simulink model "Validation_Tricopter_Model"  (R2015a)
settings: Solver=ode3  SolverMode=SingleTasking  StartTime=0.0  StopTime=20  FixedStep=T_sim  RelTol=1e-3
PreLoadFcn:
  | LoadLibraries
values from neighbouring files (symbols this model uses):
  a = 10.26    [SetupComplete.m]
  A_x = 0.015    [SetupComplete.m]
  A_y = A_x    (= 0.015)    [SetupComplete.m]
  A_z = 0.16    [SetupComplete.m]
  C_d0 = 0.001193    [SetupComplete.m]
  C_x = 1.2    [SetupComplete.m]
  C_y = C_x    (= 1.2)    [SetupComplete.m]
  C_z = 2.2    [SetupComplete.m]
  CG_0 = [0,0,0.02]'    [SetupComplete.m]
  g = 9.81    [SetupComplete.m]
  h = 0.08    [SetupComplete.m]
  h_FA = 0.02    [SetupComplete.m]
  h_M = 0.064    [SetupComplete.m]
  I_BAC_0 = [ Ix,0,Ixz;0,Iy,0;Ixz,0,Iz]    [SetupComplete.m]
  I_prop = 1/4*M_eq*R^2*diag([1,1,2])    [SetupComplete.m]
  I_tube = [1/2*M_tube*R_tube_eq^2,0,  0  ;           0 ,1/3*M_tube*l_arm^2,0;             0  ,0,1/3*M_tube*l_arm^2]    [SetupComplete.m]
  Initial_Omegas = [1;1;1]*Omega_hover    [Run3Copter.m]
  J_FA = I_prop(1,1) + m_prop*h^2  + m_FA*h_FA^2 + m_M*h_M^2    [SetupComplete.m]
  J_T = J_m+1/2*M_eq*R^2    (= 2.000642e-05)    [SetupComplete.m]
  Ki = lqi(LM_4DOF_aug, Q,R)    [robust_controller.m]
  l = 0.3450    (= 0.345)    [NDI_components.m]    (also in SetupComplete.m; robust_controller.m)
  l_arm = 0.264    [SetupComplete.m]
  m = 3.51    [SetupComplete.m]
  m_0 = 2.61    [SetupComplete.m]
  m_FA = 0.02    [SetupComplete.m]
  m_M = 0.300    (= 0.3)    [SetupComplete.m]
  m_prop = 0.02    [SetupComplete.m]
  R = 0.1778    [SetupComplete.m]    (also in robust_controller.m = eye(4))
  rho = 1.15    [SetupComplete.m]
  sigma = b*c/(pi*R)    (= 0.107416159567)    [SetupComplete.m]
  T_sim = 0.01    [Run3Copter.m]
  theta_0 = 0.38397    [SetupComplete.m]
  theta_1 = -0.2967    [SetupComplete.m]
  trim_simplemodel = [0.589627915568 -2.20656039197 0 0.588313336084 0 0 0.588313330414 0 0]    [trimvalues.mat]
  V_4DOF_last = [0.0122475086001 0.00870447045314 -0.0292257707267 -0.0198753669721 -0.00290766514824 -0.0269511839788 0.0344308792695 -0.0305235710433 -0.0274078219028 -0.0329291952852 -0.0272335702183 -0.00643013158961 ... (1500 elements, 50x30)]    [NN_c_weights.mat]
  v_i0 = sqrt( 1/3*m*g/(2*rho*pi*R^2)  )    [SetupComplete.m]
  W_4DOF_last = [0.0132359246225 -0.0402459595001 -0.0221501781133 0.0046881519205 0.0457506835434 0.0464888535199 -0.0342386918322 0.0470592781761 0.0457166948243 -0.00146243512772 0.0300280468889 -0.0358113661373 ... (204 elements, 4x51)]    [NN_c_weights.mat]
undefined symbols (not defined in the file or in its folder): DOWN_0, EAST_0, Motor, NORTH_0, P_0, Prop, Q_0, R_0, sigmatest, U_0, V_0, v_i_adim, Vx_adim, Vz_adim, W_0
undefined symbols (not defined in the file): Initial_Torques, Rotation_sign, Tau_motors
libraries: simulink x66, XXCopter x32, vrlib x26, simulink_extras x6, Adaptive_FaultTolerantControl x6, qcatlib x4, dspinverses x4, lib_controller x4, aerolib6dofsys x3, aerolibtransform2 x3, aerolib6dof2 x1
(part 2 of 11)

== system Validation_Tricopter_Model/Controller/4DOF PID Controller/4DOF PI Angle Controller ==
  note: This DCM is Tb->e
      | Xbody = DCM x Xearth
  note: Proportional controller around the hovering point. Body rates will be very similar to euler rates.
  note: INNER RATE LOOP TUNING
  note: INNER ANGLE LOOP TUNING
  measurements : Inport
  earth_ref : Inport  Port=2
  trim_control_input : Inport  Port=3
  Reference_attitude : Inport  Port=4
  Bus Selector : BusSelector  OutputSignals=euler,euler_dot,X_e,DCM,V_b
  Demux{,1,3..8} (8 alike) : Demux  Outputs=3
  Earth to body : Product  Multiplication=Matrix(*)
  Inner Rate Controller1 : ModelReference  ModelNameDialog=Inner_Rate_Controller  SimulationMode=Normal  ModelReferenceVersion=1.1241  CopyOfModelName=Inner_Rate_Controller
  Mux1 : Mux  Inputs=3
  Mux2 : Mux  Inputs=3
  Mux3 : Mux  Inputs=3
  PID Controller : simulink/Continuous/PID Controller  Controller=PI  TimeDomain=Continuous-time  SampleTime=-1  IntegratorMethod=Forward Euler  FilterMethod=Forward Euler  Form=Parallel  UseFilter=on  ControllerParametersSource=internal  P=1  I=1  D=0  N=100  InitialConditionSource=internal  InitialConditionForIntegrator=0  InitialConditionForFilter=0  ExternalReset=none  LimitOutput=off  UpperSaturationLimit=inf  LowerSaturationLimit=-inf  LinearizeAsGain=on  AntiWindupMode=none  Kb=1  TrackingMode=off  Kt=1  PParamMin=[]  PParamMax=[]  IParamMin=[]  IParamMax=[]  DParamMin=[]  DParamMax=[]  NParamMin=[]  NParamMax=[]  KbParamMin=[]  KbParamMax=[]  KtParamMin=[]  KtParamMax=[]  POutMin=[]  POutMax=[]  IOutMin=[]  IOutMax=[]  DOutMin=[]  DOutMax=[]  NOutMin=[]  NOutMax=[]  KbOutMin=[]  KbOutMax=[]  KtOutMin=[]  KtOutMax=[]  IntegratorOutMin=[]  IntegratorOutMax=[]  FilterOutMin=[]  FilterOutMax=[]  SumOutMin=[]  SumOutMax=[]  SumI1OutMin=[]  SumI1OutMax=[]  SumI2OutMin=[]  SumI2OutMax=[]  SumI3OutMin=[]  SumI3OutMax=[]  SumDOutMin=[]  SumDOutMax=[]  SaturationOutMin=[]  SaturationOutMax=[]  IntegratorContinuousStateAttributes=''  IntegratorStateMustResolveToSignalObject=off  IntegratorRTWStateStorageClass=Auto  FilterContinuousStateAttributes=''  FilterStateMustResolveToSignalObject=off  FilterRTWStateStorageClass=Auto  DifferentiatorICPrevScaledInput=0  DifferentiatorOutMin=[]  DifferentiatorOutMax=[]
  PID Controller1 : simulink/Continuous/PID Controller  Controller=PI  TimeDomain=Continuous-time  SampleTime=-1  IntegratorMethod=Forward Euler  FilterMethod=Forward Euler  Form=Parallel  UseFilter=on  ControllerParametersSource=internal  P=1  I=1  D=0  N=100  InitialConditionSource=internal  InitialConditionForIntegrator=0  InitialConditionForFilter=0  ExternalReset=none  LimitOutput=off  UpperSaturationLimit=inf  LowerSaturationLimit=-inf  LinearizeAsGain=on  AntiWindupMode=none  Kb=1  TrackingMode=off  Kt=1  PParamMin=[]  PParamMax=[]  IParamMin=[]  IParamMax=[]  DParamMin=[]  DParamMax=[]  NParamMin=[]  NParamMax=[]  KbParamMin=[]  KbParamMax=[]  KtParamMin=[]  KtParamMax=[]  POutMin=[]  POutMax=[]  IOutMin=[]  IOutMax=[]  DOutMin=[]  DOutMax=[]  NOutMin=[]  NOutMax=[]  KbOutMin=[]  KbOutMax=[]  KtOutMin=[]  KtOutMax=[]  IntegratorOutMin=[]  IntegratorOutMax=[]  FilterOutMin=[]  FilterOutMax=[]  SumOutMin=[]  SumOutMax=[]  SumI1OutMin=[]  SumI1OutMax=[]  SumI2OutMin=[]  SumI2OutMax=[]  SumI3OutMin=[]  SumI3OutMax=[]  SumDOutMin=[]  SumDOutMax=[]  SaturationOutMin=[]  SaturationOutMax=[]  IntegratorContinuousStateAttributes=''  IntegratorStateMustResolveToSignalObject=off  IntegratorRTWStateStorageClass=Auto  FilterContinuousStateAttributes=''  FilterStateMustResolveToSignalObject=off  FilterRTWStateStorageClass=Auto  DifferentiatorICPrevScaledInput=0  DifferentiatorOutMin=[]  DifferentiatorOutMax=[]
  PID Controller2 : simulink/Continuous/PID Controller  Controller=PI  TimeDomain=Continuous-time  SampleTime=-1  IntegratorMethod=Forward Euler  FilterMethod=Forward Euler  Form=Parallel  UseFilter=on  ControllerParametersSource=internal  P=1  I=0.1  D=0  N=100  InitialConditionSource=internal  InitialConditionForIntegrator=0  InitialConditionForFilter=0  ExternalReset=none  LimitOutput=off  UpperSaturationLimit=inf  LowerSaturationLimit=-inf  LinearizeAsGain=on  AntiWindupMode=none  Kb=1  TrackingMode=off  Kt=1  PParamMin=[]  PParamMax=[]  IParamMin=[]  IParamMax=[]  DParamMin=[]  DParamMax=[]  NParamMin=[]  NParamMax=[]  KbParamMin=[]  KbParamMax=[]  KtParamMin=[]  KtParamMax=[]  POutMin=[]  POutMax=[]  IOutMin=[]  IOutMax=[]  DOutMin=[]  DOutMax=[]  NOutMin=[]  NOutMax=[]  KbOutMin=[]  KbOutMax=[]  KtOutMin=[]  KtOutMax=[]  IntegratorOutMin=[]  IntegratorOutMax=[]  FilterOutMin=[]  FilterOutMax=[]  SumOutMin=[]  SumOutMax=[]  SumI1OutMin=[]  SumI1OutMax=[]  SumI2OutMin=[]  SumI2OutMax=[]  SumI3OutMin=[]  SumI3OutMax=[]  SumDOutMin=[]  SumDOutMax=[]  SaturationOutMin=[]  SaturationOutMax=[]  IntegratorContinuousStateAttributes=''  IntegratorStateMustResolveToSignalObject=off  IntegratorRTWStateStorageClass=Auto  FilterContinuousStateAttributes=''  FilterStateMustResolveToSignalObject=off  FilterRTWStateStorageClass=Auto  DifferentiatorICPrevScaledInput=0  DifferentiatorOutMin=[]  DifferentiatorOutMax=[]
  Sum : Sum  Inputs=|+-
  Sum1 : Sum  Inputs=-+|
  Sum2 : Sum  Inputs=|++
  Sum3 : Sum  Inputs=-+|
  Sum4 : Sum  Inputs=|+-
  euler_ref : Constant  Value=[0,0,0]
  Controller output : Outport
  wires:
  [psi_error] -> PID Controller2/1
  [theta_error] -> PID Controller1/1
  PID Controller2/1 -> [r_ref]
  PID Controller1/1 -> [q_ref]
  PID Controller/1 -> [p_ref]
  [phi_error] -> PID Controller/1
  Demux3/3 -> [r]
  Demux3/2 -> [q]
  Demux3/1 -> [p]
  measurements/1 -> Bus Selector/1
  Sum2/1 -> Controller output/1
  Bus Selector/2 -> Demux3/1, Sum1/1  "<euler_dot>"
  Sum1/1 -> Demux/1
  Demux/3 -> [r_error]
  Demux/2 -> [q_error]
  Demux/1 -> [p_error]
  trim_control_input/1 -> [trimmed_input]
  [trimmed_input] -> Sum2/2
  Mux2/1 -> Sum1/2
  [q_ref] -> Mux2/2
  [p_ref] -> Mux2/1
  [r_ref] -> Mux2/3
  Inner Rate Controller1/1 -> Sum2/1
  [p_error] -> Inner Rate Controller1/1
  [q_error] -> Inner Rate Controller1/2
  [r_error] -> Inner Rate Controller1/3
  Bus Selector/3 -> Demux5/1, Sum3/1  "<X_e>"
  Demux5/3 -> [Z_earth]
  Demux5/2 -> [Y_earth]
  Demux5/1 -> [X_earth]
  Demux4/3 -> [z_error]
  Demux4/2 -> [y_error]
  Demux4/1 -> [x_error]
  Mux1/1 -> Sum3/2
  [Yearth_ref] -> Mux1/2
  [Xearth_ref] -> Mux1/1
  [Zearth_ref] -> Mux1/3
  Mux3/1 -> Sum4/1
  Demux7/1 -> [vx_b]
  Demux7/2 -> [vy_b]
  Demux7/3 -> [vz_b]
  Bus Selector/5 -> Demux7/1, Sum4/2  "<V_b>"
  Sum4/1 -> Demux6/1
  Demux6/1 -> [vx_error]
  Demux6/2 -> [vy_error]
  Demux6/3 -> [vz_error]
  [Vy_body_ref] -> Mux3/2
  [Vx_body_ref] -> Mux3/1
  [Vz_body_ref] -> Mux3/3
  Bus Selector/4 -> Earth to body/2  "<DCM>"
  Earth to body/1 -> Demux4/1
  Sum3/1 -> Earth to body/1
  Demux8/3 -> [Zearth_ref]
  Demux8/2 -> [Yearth_ref]
  Demux8/1 -> [Xearth_ref]
  earth_ref/1 -> Demux8/1
  Bus Selector/1 -> Sum/2  "<euler>"
  Sum/1 -> Demux1/1
  Demux1/1 -> [phi_error]
  Demux1/2 -> [theta_error]
  Demux1/3 -> [psi_error]
  euler_ref/1 -> Sum/1

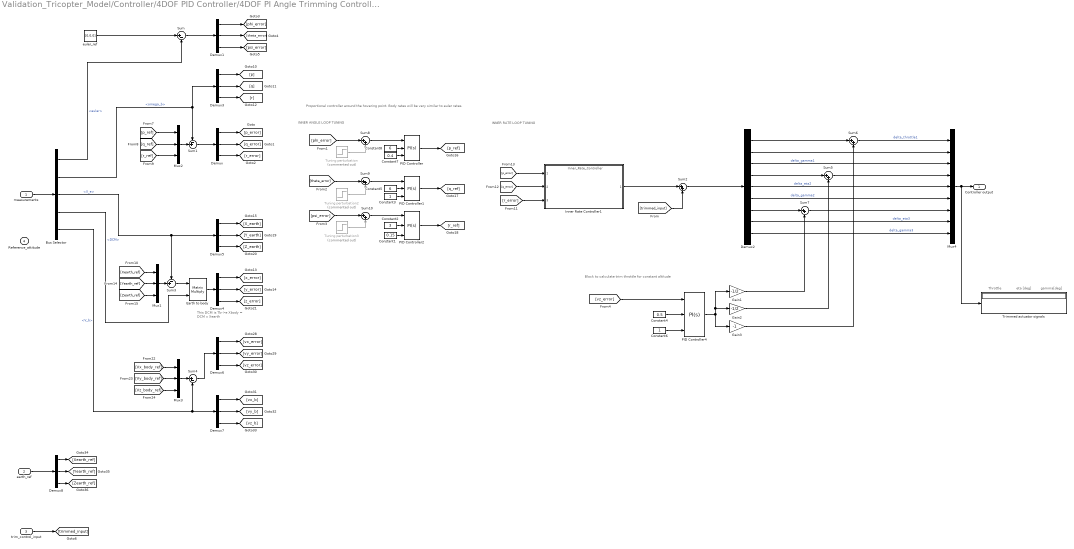
== system Validation_Tricopter_Model/Controller/4DOF PID Controller/4DOF PI Angle Trimming Controller ==
  note: Throttle
  note: Block to calculate trim throttle for constant altitude
  note: INNER ANGLE LOOP TUNING
  note: INNER RATE LOOP TUNING
  note: Proportional controller around the hovering point. Body rates will be very similar to euler rates.
  note: This DCM is Tb->e
      | Xbody = DCM x Xearth
  note: eta [deg]
  note: gamma[deg]
  measurements : Inport
  earth_ref : Inport  Port=2
  trim_control_input : Inport  Port=3
  Reference_attitude : Inport  Port=4
  Bus Selector : BusSelector  OutputSignals=euler,omega_b,X_e,DCM,V_b
  Constant1 : Constant  Value=0.15
  Constant2 : Constant  Value=3
  Constant3 : Constant
  Constant4 : Constant  Value=0.5
  Constant5 : Constant  Value=6
  Constant6 : Constant
  Constant7 : Constant  Value=0.4
  Constant8 : Constant  Value=6
  Demux{,1,3..8} (8 alike) : Demux  Outputs=3
  Demux2 : Demux  Outputs=9
  Earth to body : Product  Multiplication=Matrix(*)
  Gain1 : Gain  Gain=-1/2
  Gain2 : Gain  Gain=-1/2
  Gain3 : Gain  Gain=-1
  Inner Rate Controller1 : ModelReference  ModelNameDialog=Inner_Rate_Controller  SimulationMode=Normal  ModelReferenceVersion=1.1241  CopyOfModelName=Inner_Rate_Controller
  Mux1 : Mux  Inputs=3
  Mux2 : Mux  Inputs=3
  Mux3 : Mux  Inputs=3
  Mux4 : Mux  Inputs=9
  PID Controller : simulink/Continuous/PID Controller  Controller=PI  TimeDomain=Continuous-time  SampleTime=-1  IntegratorMethod=Forward Euler  FilterMethod=Forward Euler  Form=Parallel  UseFilter=on  ControllerParametersSource=external  P=1  I=1  D=0  N=100  InitialConditionSource=internal  InitialConditionForIntegrator=0  InitialConditionForFilter=0  ExternalReset=none  LimitOutput=off  UpperSaturationLimit=inf  LowerSaturationLimit=-inf  LinearizeAsGain=on  AntiWindupMode=none  Kb=1  TrackingMode=off  Kt=1  PParamMin=[]  PParamMax=[]  IParamMin=[]  IParamMax=[]  DParamMin=[]  DParamMax=[]  NParamMin=[]  NParamMax=[]  KbParamMin=[]  KbParamMax=[]  KtParamMin=[]  KtParamMax=[]  POutMin=[]  POutMax=[]  IOutMin=[]  IOutMax=[]  DOutMin=[]  DOutMax=[]  NOutMin=[]  NOutMax=[]  KbOutMin=[]  KbOutMax=[]  KtOutMin=[]  KtOutMax=[]  IntegratorOutMin=[]  IntegratorOutMax=[]  FilterOutMin=[]  FilterOutMax=[]  SumOutMin=[]  SumOutMax=[]  SumI1OutMin=[]  SumI1OutMax=[]  SumI2OutMin=[]  SumI2OutMax=[]  SumI3OutMin=[]  SumI3OutMax=[]  SumDOutMin=[]  SumDOutMax=[]  SaturationOutMin=[]  SaturationOutMax=[]  IntegratorContinuousStateAttributes=''  IntegratorStateMustResolveToSignalObject=off  IntegratorRTWStateStorageClass=Auto  FilterContinuousStateAttributes=''  FilterStateMustResolveToSignalObject=off  FilterRTWStateStorageClass=Auto  DifferentiatorICPrevScaledInput=0  DifferentiatorOutMin=[]  DifferentiatorOutMax=[]
  PID Controller1 : simulink/Continuous/PID Controller  Controller=PI  TimeDomain=Continuous-time  SampleTime=-1  IntegratorMethod=Forward Euler  FilterMethod=Forward Euler  Form=Parallel  UseFilter=on  ControllerParametersSource=external  P=1  I=1  D=0  N=100  InitialConditionSource=internal  InitialConditionForIntegrator=0  InitialConditionForFilter=0  ExternalReset=none  LimitOutput=off  UpperSaturationLimit=inf  LowerSaturationLimit=-inf  LinearizeAsGain=on  AntiWindupMode=none  Kb=1  TrackingMode=off  Kt=1  PParamMin=[]  PParamMax=[]  IParamMin=[]  IParamMax=[]  DParamMin=[]  DParamMax=[]  NParamMin=[]  NParamMax=[]  KbParamMin=[]  KbParamMax=[]  KtParamMin=[]  KtParamMax=[]  POutMin=[]  POutMax=[]  IOutMin=[]  IOutMax=[]  DOutMin=[]  DOutMax=[]  NOutMin=[]  NOutMax=[]  KbOutMin=[]  KbOutMax=[]  KtOutMin=[]  KtOutMax=[]  IntegratorOutMin=[]  IntegratorOutMax=[]  FilterOutMin=[]  FilterOutMax=[]  SumOutMin=[]  SumOutMax=[]  SumI1OutMin=[]  SumI1OutMax=[]  SumI2OutMin=[]  SumI2OutMax=[]  SumI3OutMin=[]  SumI3OutMax=[]  SumDOutMin=[]  SumDOutMax=[]  SaturationOutMin=[]  SaturationOutMax=[]  IntegratorContinuousStateAttributes=''  IntegratorStateMustResolveToSignalObject=off  IntegratorRTWStateStorageClass=Auto  FilterContinuousStateAttributes=''  FilterStateMustResolveToSignalObject=off  FilterRTWStateStorageClass=Auto  DifferentiatorICPrevScaledInput=0  DifferentiatorOutMin=[]  DifferentiatorOutMax=[]
  PID Controller2 : simulink/Continuous/PID Controller  Controller=PI  TimeDomain=Continuous-time  SampleTime=-1  IntegratorMethod=Forward Euler  FilterMethod=Forward Euler  Form=Parallel  UseFilter=on  ControllerParametersSource=external  P=1  I=1  D=0  N=100  InitialConditionSource=internal  InitialConditionForIntegrator=0  InitialConditionForFilter=0  ExternalReset=none  LimitOutput=off  UpperSaturationLimit=inf  LowerSaturationLimit=-inf  LinearizeAsGain=on  AntiWindupMode=none  Kb=1  TrackingMode=off  Kt=1  PParamMin=[]  PParamMax=[]  IParamMin=[]  IParamMax=[]  DParamMin=[]  DParamMax=[]  NParamMin=[]  NParamMax=[]  KbParamMin=[]  KbParamMax=[]  KtParamMin=[]  KtParamMax=[]  POutMin=[]  POutMax=[]  IOutMin=[]  IOutMax=[]  DOutMin=[]  DOutMax=[]  NOutMin=[]  NOutMax=[]  KbOutMin=[]  KbOutMax=[]  KtOutMin=[]  KtOutMax=[]  IntegratorOutMin=[]  IntegratorOutMax=[]  FilterOutMin=[]  FilterOutMax=[]  SumOutMin=[]  SumOutMax=[]  SumI1OutMin=[]  SumI1OutMax=[]  SumI2OutMin=[]  SumI2OutMax=[]  SumI3OutMin=[]  SumI3OutMax=[]  SumDOutMin=[]  SumDOutMax=[]  SaturationOutMin=[]  SaturationOutMax=[]  IntegratorContinuousStateAttributes=''  IntegratorStateMustResolveToSignalObject=off  IntegratorRTWStateStorageClass=Auto  FilterContinuousStateAttributes=''  FilterStateMustResolveToSignalObject=off  FilterRTWStateStorageClass=Auto  DifferentiatorICPrevScaledInput=0  DifferentiatorOutMin=[]  DifferentiatorOutMax=[]
  PID Controller4 : simulink/Continuous/PID Controller  Controller=PI  TimeDomain=Continuous-time  SampleTime=-1  IntegratorMethod=Forward Euler  FilterMethod=Forward Euler  Form=Parallel  UseFilter=on  ControllerParametersSource=external  P=2  I=0.5  D=0  N=100  InitialConditionSource=internal  InitialConditionForIntegrator=0  InitialConditionForFilter=0  ExternalReset=none  LimitOutput=off  UpperSaturationLimit=inf  LowerSaturationLimit=-inf  LinearizeAsGain=on  AntiWindupMode=none  Kb=1  TrackingMode=off  Kt=1  PParamMin=[]  PParamMax=[]  IParamMin=[]  IParamMax=[]  DParamMin=[]  DParamMax=[]  NParamMin=[]  NParamMax=[]  KbParamMin=[]  KbParamMax=[]  KtParamMin=[]  KtParamMax=[]  POutMin=[]  POutMax=[]  IOutMin=[]  IOutMax=[]  DOutMin=[]  DOutMax=[]  NOutMin=[]  NOutMax=[]  KbOutMin=[]  KbOutMax=[]  KtOutMin=[]  KtOutMax=[]  IntegratorOutMin=[]  IntegratorOutMax=[]  FilterOutMin=[]  FilterOutMax=[]  SumOutMin=[]  SumOutMax=[]  SumI1OutMin=[]  SumI1OutMax=[]  SumI2OutMin=[]  SumI2OutMax=[]  SumI3OutMin=[]  SumI3OutMax=[]  SumDOutMin=[]  SumDOutMax=[]  SaturationOutMin=[]  SaturationOutMax=[]  IntegratorContinuousStateAttributes=''  IntegratorStateMustResolveToSignalObject=off  IntegratorRTWStateStorageClass=Auto  FilterContinuousStateAttributes=''  FilterStateMustResolveToSignalObject=off  FilterRTWStateStorageClass=Auto  DifferentiatorICPrevScaledInput=0  DifferentiatorOutMin=[]  DifferentiatorOutMax=[]
  Sum : Sum  Inputs=|+-
  Sum1 : Sum  Inputs=-+|
  Sum{2,5..10} (7 alike) : Sum  Inputs=|++
  Sum3 : Sum  Inputs=-+|
  Sum4 : Sum  Inputs=|+-
  Trimmed actuator signals : Display
  Tuning perturbation : Step  Commented=on  Time=20  After=3*pi/180  SampleTime=0
  Tuning perturbation2 : Step  Commented=on  Time=20  After=-3*pi/180  SampleTime=0
  Tuning perturbation3 : Step  Commented=on  Time=20  After=3*pi/180  SampleTime=0
  euler_ref : Constant  Value=[0,0,0]
  Controller output : Outport
  wires:
  euler_ref/1 -> Sum/1
  Demux1/3 -> [psi_error]
  Demux1/2 -> [theta_error]
  Demux1/1 -> [phi_error]
  Sum/1 -> Demux1/1
  Bus Selector/1 -> Sum/2  "<euler>"
  earth_ref/1 -> Demux8/1
  Demux8/1 -> [Xearth_ref]
  Demux8/2 -> [Yearth_ref]
  Demux8/3 -> [Zearth_ref]
  Sum3/1 -> Earth to body/1
  Earth to body/1 -> Demux4/1
  Bus Selector/4 -> Earth to body/2  "<DCM>"
  [Vz_body_ref] -> Mux3/3
  [Vx_body_ref] -> Mux3/1
  [Vy_body_ref] -> Mux3/2
  Demux6/3 -> [vz_error]
  Demux6/2 -> [vy_error]
  Demux6/1 -> [vx_error]
  Sum4/1 -> Demux6/1
  Bus Selector/5 -> Sum4/2, Demux7/1  "<V_b>"
  Demux7/3 -> [vz_b]
  Demux7/2 -> [vy_b]
  Demux7/1 -> [vx_b]
  Mux3/1 -> Sum4/1
  [Zearth_ref] -> Mux1/3
  [Xearth_ref] -> Mux1/1
  [Yearth_ref] -> Mux1/2
  Mux1/1 -> Sum3/2
  Demux4/1 -> [x_error]
  Demux4/2 -> [y_error]
  Demux4/3 -> [z_error]
  Demux5/1 -> [X_earth]
  Demux5/2 -> [Y_earth]
  Demux5/3 -> [Z_earth]
  Bus Selector/3 -> Sum3/1, Demux5/1  "<X_e>"
  [r_error] -> Inner Rate Controller1/3
  [q_error] -> Inner Rate Controller1/2
  [p_error] -> Inner Rate Controller1/1
  Inner Rate Controller1/1 -> Sum2/1
  [r_ref] -> Mux2/3
  [p_ref] -> Mux2/1
  [q_ref] -> Mux2/2
  Mux2/1 -> Sum1/2
  [trimmed_input] -> Sum2/2
  trim_control_input/1 -> [trimmed_input]
  Demux/1 -> [p_error]
  Demux/2 -> [q_error]
  Demux/3 -> [r_error]
  Sum1/1 -> Demux/1
  Bus Selector/2 -> Sum1/1, Demux3/1  "<omega_b>"
  measurements/1 -> Bus Selector/1
  Demux3/1 -> [p]
  Demux3/2 -> [q]
  Demux3/3 -> [r]
  PID Controller/1 -> [p_ref]
  PID Controller1/1 -> [q_ref]
  PID Controller2/1 -> [r_ref]
  [vz_error] -> PID Controller4/1
  PID Controller4/1 -> Gain2/1, Gain1/1, Gain3/1
  Gain1/1 -> Sum7/2
  Gain2/1 -> Sum5/2
  Gain3/1 -> Sum6/2
  Constant4/1 -> PID Controller4/2
  Constant6/1 -> PID Controller4/3
  Sum6/1 -> Mux4/1  "delta_throttle1"
  Demux2/6 -> Mux4/6  "delta_gamma2"
  Demux2/5 -> Mux4/5  "delta_eta2"
  Demux2/3 -> Mux4/3  "delta_gamma1"
  Demux2/2 -> Mux4/2
  Demux2/9 -> Mux4/9  "delta_gamma3"
  Demux2/8 -> Mux4/8  "delta_eta3"
  Mux4/1 -> Trimmed actuator signals/1, Controller output/1
  Sum5/1 -> Mux4/4
  Sum7/1 -> Mux4/7
  Demux2/7 -> Sum7/1
  Demux2/4 -> Sum5/1
  Demux2/1 -> Sum6/1
  Sum2/1 -> Demux2/1
  Constant2/1 -> PID Controller2/2
  Constant1/1 -> PID Controller2/3
  Constant5/1 -> PID Controller1/2
  Constant8/1 -> PID Controller/2
  Constant7/1 -> PID Controller/3
  Constant3/1 -> PID Controller1/3
  Sum8/1 -> PID Controller/1
  [phi_error] -> Sum8/1
  [theta_error] -> Sum9/1
  [psi_error] -> Sum10/1
  Sum10/1 -> PID Controller2/1
  Sum9/1 -> PID Controller1/1
  Tuning perturbation3/1 -> Sum10/2
  Tuning perturbation/1 -> Sum8/2
  Tuning perturbation2/1 -> Sum9/2

== system Validation_Tricopter_Model/Controller/4DOF PID Controller/4DOF PI Rate Trimming Controller ==
  note: This block is used to calculate the trimming values for the inner loop rates
  note: INNER LOOP TUNING
  measurements : Inport
  earth_ref : Inport  Port=2
  trim_control_input : Inport  Port=3
  Reference_attitude : Inport  Port=4
  Bus Selector : BusSelector  OutputSignals=euler,euler_dot
  Demux{,1..5} (6 alike) : Demux  Outputs=3
  Euler_dot_ref : Constant  Value=[0 0 0]
  Euler_ref : Constant  Value=[0 0 0]
  Inner Rate Controller : ModelReference  ModelNameDialog=Inner_Rate_Controller  SimulationMode=Normal  ModelReferenceVersion=1.1241  CopyOfModelName=Inner_Rate_Controller
  Sum : Sum  Inputs=|+-
  Sum1 : Sum  Inputs=-+|
  Sum2 : Sum  Inputs=|++
  Controller output : Outport
  wires:
  trim_control_input/1 -> [trimmed_input]
  Demux1/3 -> [psi_error]
  Demux1/2 -> [theta_error]
  Demux1/1 -> [phi_error]
  Demux/1 -> [p_error]
  Demux/2 -> [q_error]
  Demux/3 -> [r_error]
  Sum/1 -> Demux1/1
  Sum1/1 -> Demux/1
  Bus Selector/2 -> Sum1/1, Demux3/1  "<euler_dot>"
  Bus Selector/1 -> Sum/2, Demux2/1  "<euler>"
  measurements/1 -> Bus Selector/1
  Demux2/3 -> [psi]
  Demux2/2 -> [theta]
  Demux2/1 -> [phi]
  Demux3/1 -> [p]
  Demux3/2 -> [q]
  Demux3/3 -> [r]
  Demux4/3 -> [psi_ref]
  Demux4/2 -> [theta_ref]
  Demux4/1 -> [phi_ref]
  Euler_ref/1 -> Demux4/1, Sum/1
  Demux5/1 -> [p_ref]
  Demux5/2 -> [q_ref]
  Demux5/3 -> [r_ref]
  Euler_dot_ref/1 -> Demux5/1, Sum1/2
  [r_error] -> Inner Rate Controller/3
  [p_error] -> Inner Rate Controller/1
  [q_error] -> Inner Rate Controller/2
  Inner Rate Controller/1 -> Sum2/1
  Sum2/1 -> Controller output/1
  [trimmed_input] -> Sum2/2

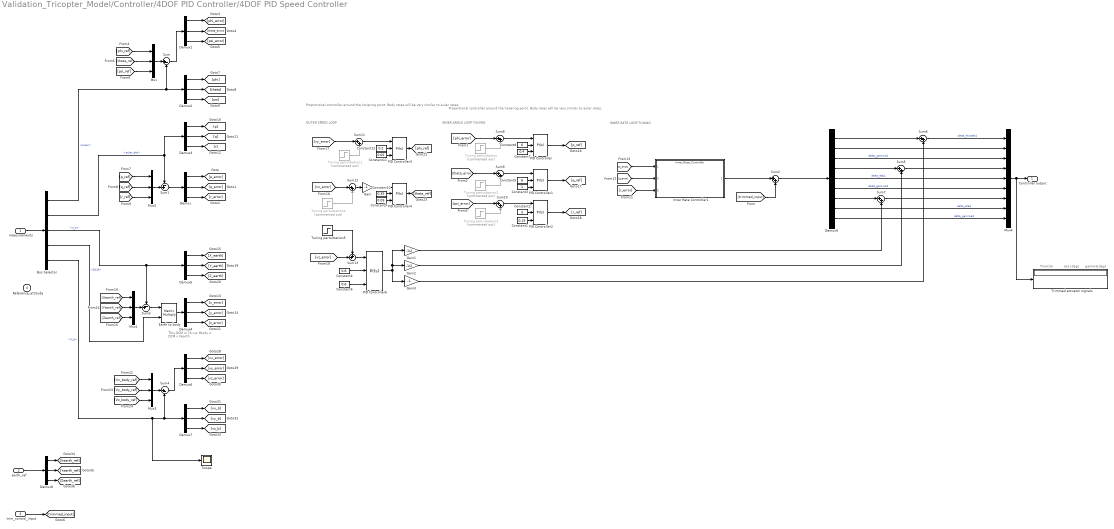
== system Validation_Tricopter_Model/Controller/4DOF PID Controller/4DOF PID Speed Controller ==
  note: This DCM is Tb->e
      | Xbody = DCM x Xearth
  note: Proportional controller around the hovering point. Body rates will be very similar to euler rates.
  note: OUTER SPEED LOOP
  note: Throttle
  note: INNER ANGLE LOOP TUNING
  note: INNER RATE LOOP TUNING
  note: Proportional controller around the hovering point. Body rates will be very similar to euler rates.
  note: eta [deg]
  note: gamma[deg]
  measurements : Inport
  earth_ref : Inport  Port=2
  trim_control_input : Inport  Port=3
  Reference_attitude : Inport  Port=4
  Bus Selector : BusSelector  OutputSignals=euler,euler_dot,X_e,DCM,V_b
  Constant1 : Constant  Value=0.15
  Constant10 : Constant  Value=0.35
  Constant11 : Constant  Value=0.02
  Constant12 : Constant  Value=0.2
  Constant2 : Constant  Value=3
  Constant3 : Constant
  Constant4 : Constant  Value=0.8
  Constant5 : Constant  Value=6
  Constant6 : Constant  Value=0.6
  Constant7 : Constant  Value=0.4
  Constant8 : Constant  Value=6
  Constant9 : Constant  Value=0.03
  Demux{,1..8} (9 alike) : Demux  Outputs=3
  Demux9 : Demux  Outputs=9
  Earth to body : Product  Multiplication=Matrix(*)
  Gain : Gain  Gain=-1
  Gain1 : Gain  Gain=-1/2
  Gain2 : Gain  Gain=-1/2
  Gain3 : Gain  Gain=-1
  Inner Rate Controller1 : ModelReference  ModelNameDialog=Inner_Rate_Controller  SimulationMode=Normal  ModelReferenceVersion=1.1241  CopyOfModelName=Inner_Rate_Controller
  Mux{,1..3} (4 alike) : Mux  Inputs=3
  Mux4 : Mux  Inputs=9
  PID Controller{,1..4} (5 alike) : simulink/Continuous/PID Controller  Controller=PI  TimeDomain=Continuous-time  SampleTime=-1  IntegratorMethod=Forward Euler  FilterMethod=Forward Euler  Form=Parallel  UseFilter=on  ControllerParametersSource=external  P=1  I=1  D=0  N=100  InitialConditionSource=internal  InitialConditionForIntegrator=0  InitialConditionForFilter=0  ExternalReset=none  LimitOutput=off  UpperSaturationLimit=inf  LowerSaturationLimit=-inf  LinearizeAsGain=on  AntiWindupMode=none  Kb=1  TrackingMode=off  Kt=1  PParamMin=[]  PParamMax=[]  IParamMin=[]  IParamMax=[]  DParamMin=[]  DParamMax=[]  NParamMin=[]  NParamMax=[]  KbParamMin=[]  KbParamMax=[]  KtParamMin=[]  KtParamMax=[]  POutMin=[]  POutMax=[]  IOutMin=[]  IOutMax=[]  DOutMin=[]  DOutMax=[]  NOutMin=[]  NOutMax=[]  KbOutMin=[]  KbOutMax=[]  KtOutMin=[]  KtOutMax=[]  IntegratorOutMin=[]  IntegratorOutMax=[]  FilterOutMin=[]  FilterOutMax=[]  SumOutMin=[]  SumOutMax=[]  SumI1OutMin=[]  SumI1OutMax=[]  SumI2OutMin=[]  SumI2OutMax=[]  SumI3OutMin=[]  SumI3OutMax=[]  SumDOutMin=[]  SumDOutMax=[]  SaturationOutMin=[]  SaturationOutMax=[]  IntegratorContinuousStateAttributes=''  IntegratorStateMustResolveToSignalObject=off  IntegratorRTWStateStorageClass=Auto  FilterContinuousStateAttributes=''  FilterStateMustResolveToSignalObject=off  FilterRTWStateStorageClass=Auto  DifferentiatorICPrevScaledInput=0  DifferentiatorOutMin=[]  DifferentiatorOutMax=[]
  PID Controller6 : simulink/Continuous/PID Controller  Controller=PI  TimeDomain=Continuous-time  SampleTime=-1  IntegratorMethod=Forward Euler  FilterMethod=Forward Euler  Form=Parallel  UseFilter=on  ControllerParametersSource=external  P=2  I=0.5  D=0  N=100  InitialConditionSource=internal  InitialConditionForIntegrator=0  InitialConditionForFilter=0  ExternalReset=none  LimitOutput=off  UpperSaturationLimit=inf  LowerSaturationLimit=-inf  LinearizeAsGain=on  AntiWindupMode=none  Kb=1  TrackingMode=off  Kt=1  PParamMin=[]  PParamMax=[]  IParamMin=[]  IParamMax=[]  DParamMin=[]  DParamMax=[]  NParamMin=[]  NParamMax=[]  KbParamMin=[]  KbParamMax=[]  KtParamMin=[]  KtParamMax=[]  POutMin=[]  POutMax=[]  IOutMin=[]  IOutMax=[]  DOutMin=[]  DOutMax=[]  NOutMin=[]  NOutMax=[]  KbOutMin=[]  KbOutMax=[]  KtOutMin=[]  KtOutMax=[]  IntegratorOutMin=[]  IntegratorOutMax=[]  FilterOutMin=[]  FilterOutMax=[]  SumOutMin=[]  SumOutMax=[]  SumI1OutMin=[]  SumI1OutMax=[]  SumI2OutMin=[]  SumI2OutMax=[]  SumI3OutMin=[]  SumI3OutMax=[]  SumDOutMin=[]  SumDOutMax=[]  SaturationOutMin=[]  SaturationOutMax=[]  IntegratorContinuousStateAttributes=''  IntegratorStateMustResolveToSignalObject=off  IntegratorRTWStateStorageClass=Auto  FilterContinuousStateAttributes=''  FilterStateMustResolveToSignalObject=off  FilterRTWStateStorageClass=Auto  DifferentiatorICPrevScaledInput=0  DifferentiatorOutMin=[]  DifferentiatorOutMax=[]
  Scope : Scope
      settings: YMin=-1.1  YMax=0.8  SaveName=ScopeData7
  Sum : Sum  Inputs=|+-
  Sum1 : Sum  Inputs=-+|
  Sum{2,5..12} (9 alike) : Sum  Inputs=|++
  Sum13 : Sum  Inputs=++|
  Sum3 : Sum  Inputs=-+|
  Sum4 : Sum  Inputs=|+-
  Trimmed actuator signals : Display
  Tuning perturbation : Step  Commented=on  Time=20  After=3*pi/180  SampleTime=0
  Tuning perturbation1 : Step  Commented=on  Time=20  SampleTime=0
  Tuning perturbation2 : Step  Commented=on  Time=20  After=-3*pi/180  SampleTime=0
  Tuning perturbation3 : Step  Commented=on  Time=20  After=3*pi/180  SampleTime=0
  Tuning perturbation4 : Step  Commented=on  Time=20  SampleTime=0
  Tuning perturbation5 : Step  Time=20  After=-1  SampleTime=0
  Controller output : Outport
  wires:
  Mux/1 -> Sum/1
  Demux3/3 -> [r]
  Demux3/2 -> [q]
  Demux3/1 -> [p]
  Demux2/1 -> [phi]
  Demux2/2 -> [theta]
  Demux2/3 -> [psi]
  measurements/1 -> Bus Selector/1
  Bus Selector/1 -> Demux2/1, Sum/2  "<euler>"
  Bus Selector/2 -> Demux3/1, Sum1/1  "<euler_dot>"
  Sum1/1 -> Demux/1
  Sum/1 -> Demux1/1
  Demux/3 -> [r_error]
  Demux/2 -> [q_error]
  Demux/1 -> [p_error]
  Demux1/1 -> [phi_error]
  Demux1/2 -> [theta_error]
  Demux1/3 -> [psi_error]
  trim_control_input/1 -> [trimmed_input]
  [theta_ref] -> Mux/2
  [phi_ref] -> Mux/1
  [psi_ref] -> Mux/3
  Mux2/1 -> Sum1/2
  [q_ref] -> Mux2/2
  [p_ref] -> Mux2/1
  [r_ref] -> Mux2/3
  Bus Selector/3 -> Demux5/1, Sum3/1  "<X_e>"
  Demux5/3 -> [Z_earth]
  Demux5/2 -> [Y_earth]
  Demux5/1 -> [X_earth]
  Demux4/3 -> [z_error]
  Demux4/2 -> [y_error]
  Demux4/1 -> [x_error]
  Mux1/1 -> Sum3/2
  [Yearth_ref] -> Mux1/2
  [Xearth_ref] -> Mux1/1
  [Zearth_ref] -> Mux1/3
  Mux3/1 -> Sum4/1
  Demux7/1 -> [vx_b]
  Demux7/2 -> [vy_b]
  Demux7/3 -> [vz_b]
  Bus Selector/5 -> Scope/1, Demux7/1, Sum4/2  "<V_b>"
  Sum4/1 -> Demux6/1
  Demux6/1 -> [vx_error]
  Demux6/2 -> [vy_error]
  Demux6/3 -> [vz_error]
  [Vy_body_ref] -> Mux3/2
  [Vx_body_ref] -> Mux3/1
  [Vz_body_ref] -> Mux3/3
  Bus Selector/4 -> Earth to body/2  "<DCM>"
  Earth to body/1 -> Demux4/1
  Sum3/1 -> Earth to body/1
  Demux8/3 -> [Zearth_ref]
  Demux8/2 -> [Yearth_ref]
  Demux8/1 -> [Xearth_ref]
  earth_ref/1 -> Demux8/1
  [r_error] -> Inner Rate Controller1/3
  [q_error] -> Inner Rate Controller1/2
  [p_error] -> Inner Rate Controller1/1
  Inner Rate Controller1/1 -> Sum2/1
  [trimmed_input] -> Sum2/2
  PID Controller/1 -> [p_ref]
  PID Controller1/1 -> [q_ref]
  PID Controller2/1 -> [r_ref]
  PID Controller6/1 -> Gain2/1, Gain1/1, Gain3/1
  Gain1/1 -> Sum7/2
  Gain2/1 -> Sum5/2
  Gain3/1 -> Sum6/2
  Constant4/1 -> PID Controller6/2
  Constant6/1 -> PID Controller6/3
  Sum6/1 -> Mux4/1  "delta_throttle1"
  Demux9/6 -> Mux4/6  "delta_gamma2"
  Demux9/5 -> Mux4/5  "delta_eta2"
  Demux9/3 -> Mux4/3  "delta_gamma1"
  Demux9/2 -> Mux4/2
  Demux9/9 -> Mux4/9  "delta_gamma3"
  Demux9/8 -> Mux4/8  "delta_eta3"
  Mux4/1 -> Trimmed actuator signals/1, Controller output/1
  Sum5/1 -> Mux4/4
  Sum7/1 -> Mux4/7
  Demux9/7 -> Sum7/1
  Demux9/4 -> Sum5/1
  Demux9/1 -> Sum6/1
  Sum2/1 -> Demux9/1
  Constant2/1 -> PID Controller2/2
  Constant1/1 -> PID Controller2/3
  Constant5/1 -> PID Controller1/2
  Constant8/1 -> PID Controller/2
  Constant7/1 -> PID Controller/3
  Constant3/1 -> PID Controller1/3
  Sum8/1 -> PID Controller/1
  [phi_error] -> Sum8/1
  [theta_error] -> Sum9/1
  [psi_error] -> Sum10/1
  Sum10/1 -> PID Controller2/1
  Sum9/1 -> PID Controller1/1
  Tuning perturbation3/1 -> Sum10/2
  Tuning perturbation/1 -> Sum8/2
  Tuning perturbation2/1 -> Sum9/2
  PID Controller3/1 -> [phi_ref]
  PID Controller4/1 -> [theta_ref]
  Constant10/1 -> PID Controller4/2
  Constant12/1 -> PID Controller3/2
  Constant11/1 -> PID Controller3/3
  Constant9/1 -> PID Controller4/3
  Sum11/1 -> PID Controller3/1
  [vy_error] -> Sum11/1
  [vx_error] -> Sum12/1
  Sum12/1 -> Gain/1
  Tuning perturbation1/1 -> Sum11/2
  Tuning perturbation4/1 -> Sum12/2
  Gain/1 -> PID Controller4/1
  Tuning perturbation5/1 -> Sum13/1
  [vz_error] -> Sum13/2
  Sum13/1 -> PID Controller6/1

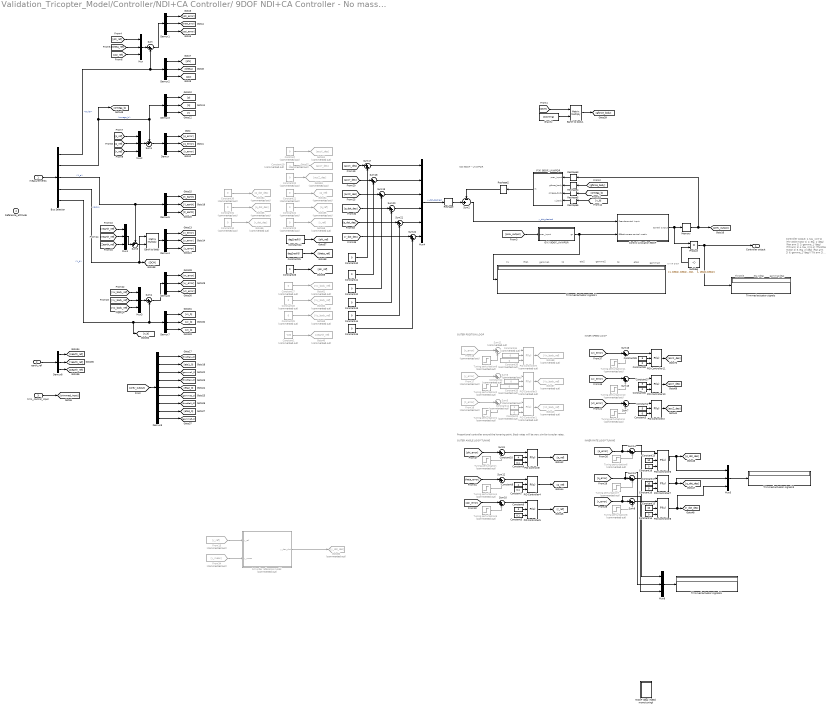
== system Validation_Tricopter_Model/Controller/NDI+CA Controller/ 9DOF NDI+CA Controller - No massic update ==
  note: gamma3
  note: gamma2
  note: gamma1
  note: eta3
  note: eta2
  note: eta1
  note: t3
  note: t2
  note: t1
  note: u
      | v
      | w
      | p
      | q
      | r
  note: OUTER POSITION LOOP
  note: gamma[deg]
  note: eta [deg]
  note: Throttle
  note: Controller output:
      | 1. tau_1 [0-1] (Thr ottle motor 1)
      | 2. eta_1 (deg)  (Pan arm 1)
      | 3. gamma_1 (deg)  (Tilt arm 1)
      |
      | 4. tau_2 [0-1] (Throttle motor 2)
      | 5. eta_2 (deg)  (Pan arm 2)
      | 6. gamma_2 (deg)  (Tilt arm 2)
      |
      | 7. tau_3 [0-1] (Throttle motor 3)
      | 8. eta_3 (deg)  (Pan arm  3)
      | 9. gamma_3 (deg)  (Tilt arm 3)
  note: Proportional controller around the hovering point. Body rates will be very similar to euler rates.
  note: INNER RATE LOOP TUNING
  note: OUTER ANGLE LOOP TUNING
  note: INNER SPEED LOOP
  note: NDI 9DOF - UVWPQR
  measurements : Inport
  earth_ref : Inport  Port=2
  trim_control_input : Inport  Port=3
  Reference_attitude : Inport  Port=4
  1st order reference model : Subsystem  Commented=on  mask(1st order model reference block){Kref=1, Kb=20, fi=0.25, fc=0.5, Kf=1}
      mask prompts: Kref "1st order reference gain"; Kb "Bandwidth gain"; fi "Integral gain"; fc "Command FF gain"; Kf "Command_dot FF gain"
      mask help:
      | Generates a desired first order derivative of a commanded output taking
      | into account the current measured output.
      | Kref is the gain that determines the first order system between y_ref and
      | y_commanded signals. Ycom/Yref = Kref/(1 + Kref)
      | fi and fc can be defaulted to 0.25 and 0.5 for a critically damped 2nd
      | order response between y_meas and the error signal (y_com - y_meas) considering
      | a perfect dynamic inversion.
      mask Help:
      | Juan Herrero Macias <jn.herrerom@gmail.com>
      | This architecture can be found and explained in Fault-tolerant Flight
      | Control and Guidance Systems, Ducard, Guillaume.
      mask TypeOptions Kref: Kref gain/Gain
      mask TypeOptions Kb: Bandwidth gain/Gain
      mask TypeOptions fi: Integral gain/Gain
      mask TypeOptions fc: Command FF gain/Gain
      mask TypeOptions Kf: Command_dot FF gain/Gain
  9 DOF Ideal (Need more tuning) : Subsystem
  Bus Selector : BusSelector  OutputSignals=euler,omega_b,X_e,DCM,V_b
  Constant{,2,12,19..23,27..35} (17 alike) : Constant  Commented=on  Value=0
  Constant1 : Constant  Commented=on  Value=-100
  Constant10 : Constant  Value=4
  Constant11 : Constant  Commented=on
  Constant13 : Constant  Value=10
  Constant{3,14,16,18,26,36,38,40..45} (13 alike) : Constant  Value=0
  Constant15 : Constant  Value=10
  Constant17 : Constant  Value=10
  Constant24 : Constant  Value=deg2rad(0)
  Constant25 : Constant  Value=deg2rad(0)
  Constant37 : Constant  Value=5
  Constant39 : Constant  Value=5
  Constant4 : Constant  Value=5
  Constant5 : Constant  Value=0.1
  Constant6 : Constant  Value=3
  Constant7 : Constant  Value=0.1
  Constant8 : Constant  Value=4
  Constant9 : Constant  Value=0.1
  Control Allocation 9DOF : Subsystem  Variant=on  OverrideUsingVariant=(default)
  Demux{,1..8} (9 alike) : Demux  Outputs=3
  Demux9 : Demux  Outputs=9
  Earth to body : Product  Multiplication=Matrix(*)
  Earth to body1 : Product  Multiplication=Matrix(*)
  F(X) 9DOF_UVWPQR : MATLAB Function  TreatAsAtomicUnit=on
  From13 : From  Commented=on  GotoTag=y_ref
  From16 : From  Commented=on  GotoTag=z_error
  From17 : From  Commented=on  GotoTag=y_error
  From18 : From  Commented=on  GotoTag=x_error
  From34 : From  Commented=on  GotoTag=y_meas
  G(X) 9DOF_UVWPQR : MATLAB Function  TreatAsAtomicUnit=on
  Goto40 : Goto  Commented=on  GotoTag=Zearth_ref
  Goto43 : Goto  Commented=on  GotoTag=Vz_body_ref
  Goto51 : Goto  Commented=on  GotoTag=accX_des
  Goto52 : Goto  Commented=on  GotoTag=accY_des
  Goto53 : Goto  Commented=on  GotoTag=accZ_des
  Goto54 : Goto  Commented=on  GotoTag=p_ref
  Goto55 : Goto  Commented=on  GotoTag=q_ref
  Goto56 : Goto  Commented=on  GotoTag=r_ref
  Goto60 : Goto  Commented=on  GotoTag=y_dot_des
  Goto61 : Goto  Commented=on  GotoTag=Vx_body_ref
  Goto62 : Goto  Commented=on  GotoTag=Vy_body_ref
  Goto63 : Goto  Commented=on  GotoTag=Vz_body_ref
  Goto64 : Goto  Commented=on  GotoTag=p_dot_des
  Goto65 : Goto  Commented=on  GotoTag=q_dot_des
  Goto66 : Goto  Commented=on  GotoTag=r_dot_des
  Goto67 : Goto  Commented=on  GotoTag=Vy_body_ref
  Goto68 : Goto  Commented=on  GotoTag=Vx_body_ref
  Gravity : Constant  Value=[0;0;m*g]
  Memory : Memory  X0=[0,0,0,0,0,0,0,0,0]  LinearizeAsDelay=on
  Mux{,1..3,5,8} (6 alike) : Mux  Inputs=3
  Mux4 : Mux  Inputs=6
  PID Controller{,2,4..8,10..11} (9 alike) : simulink/Continuous/PID Controller  Controller=PI  TimeDomain=Continuous-time  SampleTime=-1  IntegratorMethod=Forward Euler  FilterMethod=Forward Euler  Form=Parallel  UseFilter=on  ControllerParametersSource=external  P=1  I=1  D=0  N=100  InitialConditionSource=internal  InitialConditionForIntegrator=0  InitialConditionForFilter=0  ExternalReset=none  LimitOutput=off  UpperSaturationLimit=inf  LowerSaturationLimit=-inf  LinearizeAsGain=on  AntiWindupMode=none  Kb=1  TrackingMode=off  Kt=1  PParamMin=[]  PParamMax=[]  IParamMin=[]  IParamMax=[]  DParamMin=[]  DParamMax=[]  NParamMin=[]  NParamMax=[]  KbParamMin=[]  KbParamMax=[]  KtParamMin=[]  KtParamMax=[]  POutMin=[]  POutMax=[]  IOutMin=[]  IOutMax=[]  DOutMin=[]  DOutMax=[]  NOutMin=[]  NOutMax=[]  KbOutMin=[]  KbOutMax=[]  KtOutMin=[]  KtOutMax=[]  IntegratorOutMin=[]  IntegratorOutMax=[]  FilterOutMin=[]  FilterOutMax=[]  SumOutMin=[]  SumOutMax=[]  SumI1OutMin=[]  SumI1OutMax=[]  SumI2OutMin=[]  SumI2OutMax=[]  SumI3OutMin=[]  SumI3OutMax=[]  SumDOutMin=[]  SumDOutMax=[]  SaturationOutMin=[]  SaturationOutMax=[]  IntegratorContinuousStateAttributes=''  IntegratorStateMustResolveToSignalObject=off  IntegratorRTWStateStorageClass=Auto  FilterContinuousStateAttributes=''  FilterStateMustResolveToSignalObject=off  FilterRTWStateStorageClass=Auto  DifferentiatorICPrevScaledInput=0  DifferentiatorOutMin=[]  DifferentiatorOutMax=[]
  PID Controller1 : simulink/Continuous/PID Controller  Commented=on  Controller=PI  TimeDomain=Continuous-time  SampleTime=-1  IntegratorMethod=Forward Euler  FilterMethod=Forward Euler  Form=Parallel  UseFilter=on  ControllerParametersSource=external  P=1  I=1  D=0  N=100  InitialConditionSource=internal  InitialConditionForIntegrator=0  InitialConditionForFilter=0  ExternalReset=none  LimitOutput=off  UpperSaturationLimit=inf  LowerSaturationLimit=-inf  LinearizeAsGain=on  AntiWindupMode=none  Kb=1  TrackingMode=off  Kt=1  PParamMin=[]  PParamMax=[]  IParamMin=[]  IParamMax=[]  DParamMin=[]  DParamMax=[]  NParamMin=[]  NParamMax=[]  KbParamMin=[]  KbParamMax=[]  KtParamMin=[]  KtParamMax=[]  POutMin=[]  POutMax=[]  IOutMin=[]  IOutMax=[]  DOutMin=[]  DOutMax=[]  NOutMin=[]  NOutMax=[]  KbOutMin=[]  KbOutMax=[]  KtOutMin=[]  KtOutMax=[]  IntegratorOutMin=[]  IntegratorOutMax=[]  FilterOutMin=[]  FilterOutMax=[]  SumOutMin=[]  SumOutMax=[]  SumI1OutMin=[]  SumI1OutMax=[]  SumI2OutMin=[]  SumI2OutMax=[]  SumI3OutMin=[]  SumI3OutMax=[]  SumDOutMin=[]  SumDOutMax=[]  SaturationOutMin=[]  SaturationOutMax=[]  IntegratorContinuousStateAttributes=''  IntegratorStateMustResolveToSignalObject=off  IntegratorRTWStateStorageClass=Auto  FilterContinuousStateAttributes=''  FilterStateMustResolveToSignalObject=off  FilterRTWStateStorageClass=Auto  DifferentiatorICPrevScaledInput=0  DifferentiatorOutMin=[]  DifferentiatorOutMax=[]
  PID Controller3 : simulink/Continuous/PID Controller  Commented=on  Controller=PI  TimeDomain=Continuous-time  SampleTime=-1  IntegratorMethod=Forward Euler  FilterMethod=Forward Euler  Form=Parallel  UseFilter=on  ControllerParametersSource=external  P=1  I=1  D=0  N=100  InitialConditionSource=internal  InitialConditionForIntegrator=0  InitialConditionForFilter=0  ExternalReset=none  LimitOutput=off  UpperSaturationLimit=inf  LowerSaturationLimit=-inf  LinearizeAsGain=on  AntiWindupMode=none  Kb=1  TrackingMode=off  Kt=1  PParamMin=[]  PParamMax=[]  IParamMin=[]  IParamMax=[]  DParamMin=[]  DParamMax=[]  NParamMin=[]  NParamMax=[]  KbParamMin=[]  KbParamMax=[]  KtParamMin=[]  KtParamMax=[]  POutMin=[]  POutMax=[]  IOutMin=[]  IOutMax=[]  DOutMin=[]  DOutMax=[]  NOutMin=[]  NOutMax=[]  KbOutMin=[]  KbOutMax=[]  KtOutMin=[]  KtOutMax=[]  IntegratorOutMin=[]  IntegratorOutMax=[]  FilterOutMin=[]  FilterOutMax=[]  SumOutMin=[]  SumOutMax=[]  SumI1OutMin=[]  SumI1OutMax=[]  SumI2OutMin=[]  SumI2OutMax=[]  SumI3OutMin=[]  SumI3OutMax=[]  SumDOutMin=[]  SumDOutMax=[]  SaturationOutMin=[]  SaturationOutMax=[]  IntegratorContinuousStateAttributes=''  IntegratorStateMustResolveToSignalObject=off  IntegratorRTWStateStorageClass=Auto  FilterContinuousStateAttributes=''  FilterStateMustResolveToSignalObject=off  FilterRTWStateStorageClass=Auto  DifferentiatorICPrevScaledInput=0  DifferentiatorOutMin=[]  DifferentiatorOutMax=[]
  PID Controller9 : simulink/Continuous/PID Controller  Commented=on  Controller=PI  TimeDomain=Continuous-time  SampleTime=-1  IntegratorMethod=Forward Euler  FilterMethod=Forward Euler  Form=Parallel  UseFilter=on  ControllerParametersSource=external  P=1  I=1  D=0  N=100  InitialConditionSource=internal  InitialConditionForIntegrator=0  InitialConditionForFilter=0  ExternalReset=none  LimitOutput=off  UpperSaturationLimit=inf  LowerSaturationLimit=-inf  LinearizeAsGain=on  AntiWindupMode=none  Kb=1  TrackingMode=off  Kt=1  PParamMin=[]  PParamMax=[]  IParamMin=[]  IParamMax=[]  DParamMin=[]  DParamMax=[]  NParamMin=[]  NParamMax=[]  KbParamMin=[]  KbParamMax=[]  KtParamMin=[]  KtParamMax=[]  POutMin=[]  POutMax=[]  IOutMin=[]  IOutMax=[]  DOutMin=[]  DOutMax=[]  NOutMin=[]  NOutMax=[]  KbOutMin=[]  KbOutMax=[]  KtOutMin=[]  KtOutMax=[]  IntegratorOutMin=[]  IntegratorOutMax=[]  FilterOutMin=[]  FilterOutMax=[]  SumOutMin=[]  SumOutMax=[]  SumI1OutMin=[]  SumI1OutMax=[]  SumI2OutMin=[]  SumI2OutMax=[]  SumI3OutMin=[]  SumI3OutMax=[]  SumDOutMin=[]  SumDOutMax=[]  SaturationOutMin=[]  SaturationOutMax=[]  IntegratorContinuousStateAttributes=''  IntegratorStateMustResolveToSignalObject=off  IntegratorRTWStateStorageClass=Auto  FilterContinuousStateAttributes=''  FilterStateMustResolveToSignalObject=off  FilterRTWStateStorageClass=Auto  DifferentiatorICPrevScaledInput=0  DifferentiatorOutMin=[]  DifferentiatorOutMax=[]
  Product : Product
  Reshape : Reshape  OutputDimensionality=Column vector (2-D)
  Reshape2 : Reshape  OutputDimensionality=Column vector (2-D)  OutputDimensions=[6,1]
  Reshape{3..6} (4 alike) : Reshape  OutputDimensions=[6,1]
  Sum : Sum  Inputs=|+-
  Sum1 : Sum  Inputs=-+|
  Sum{7..10,12..22} (15 alike) : Sum  Inputs=|++
  Sum11 : Sum  Commented=on  Inputs=|++
  Sum2 : Sum  Inputs=-+|
  Sum3 : Sum  Inputs=-+|
  Sum4 : Sum  Inputs=|+-
  Sum5 : Sum  Commented=on  Inputs=|++
  Sum6 : Sum  Commented=on  Inputs=|++
  Trimmed actuator signals{,1,3,5} (4 alike) : Display
  Tuning perturbation{,5..6,8} (4 alike) : Step  Commented=on  Time=20  After=3*pi/180  SampleTime=0
  Tuning perturbation{1..3,9..11} (6 alike) : Step  Commented=on  Time=20  SampleTime=0
  Tuning perturbation4 : Step  Commented=on  Time=20  After=-3*pi/180  SampleTime=0
  Tuning perturbation7 : Step  Commented=on  Time=20  After=-3*pi/180  SampleTime=0
  rad2deg : Constant  Value="[1, 180/pi, 180/pi,    1,180/pi, 180/pi,     1, 180/pi,180/pi]"
  Controller output : Outport
  wires:
  PID Controller9/1 -> Goto68/1
  Tuning perturbation9/1 -> Sum11/2
  From18/1 -> Sum11/1
  Sum11/1 -> PID Controller9/1
  Constant35/1 -> PID Controller9/3
  Constant34/1 -> PID Controller9/2
  PID Controller3/1 -> Goto67/1
  Tuning perturbation2/1 -> Sum6/2
  From17/1 -> Sum6/1
  Sum6/1 -> PID Controller3/1
  Constant33/1 -> PID Controller3/3
  Constant12/1 -> PID Controller3/2
  PID Controller1/1 -> Goto43/1
  Tuning perturbation1/1 -> Sum5/2
  Sum5/1 -> PID Controller1/1
  Constant2/1 -> PID Controller1/3
  Constant11/1 -> PID Controller1/2
  Constant1/1 -> Goto40/1
  G(X) 9DOF_UVWPQR/1(gx) -> Trimmed actuator signals1/1, Control Allocation 9DOF/2(Effectiveness control matrix)
  [prev_output] -> G(X) 9DOF_UVWPQR/1(prev_input)
  Control Allocation 9DOF/1(Control output) -> Memory/1, Product/1
  Sum2/1 -> Control Allocation 9DOF/1(Pseudocontrol input)  "y_dot_desired"
  Constant13/1 -> PID Controller6/2
  Sum3/1 -> Earth to body/2
  Constant32/1 -> Goto66/1
  Constant31/1 -> Goto65/1
  Constant30/1 -> Goto64/1
  Memory/1 -> [prev_output], Reshape3/1
  [DCM] -> Earth to body1/1
  Mux8/1 -> Trimmed actuator signals5/1
  [r_error] -> Sum8/1, Mux8/3
  [q_error] -> Sum13/1, Mux8/2
  [p_error] -> Sum14/1, Mux8/1
  [psi_error] -> Sum10/1
  [theta_error] -> Sum12/1
  [phi_error] -> Sum9/1
  Constant29/1 -> Goto63/1
  Constant28/1 -> Goto62/1
  Constant27/1 -> Goto61/1
  PID Controller2/1 -> [accZ_des]
  Mux5/1 -> Trimmed actuator signals3/1
  1st order reference model/1(y_des_dot) -> Goto60/1
  From34/1 -> 1st order reference model/2(y_meas)
  From13/1 -> 1st order reference model/1(y_ref)
  rad2deg/1 -> Product/2
  Product/1 -> Controller output/1, Trimmed actuator signals/1
  Constant18/1 -> PID Controller6/3
  Constant26/1 -> [psi_ref]
  Constant25/1 -> [theta_ref]
  Constant24/1 -> [phi_ref]
  Constant23/1 -> Goto56/1
  Constant22/1 -> Goto55/1
  Constant21/1 -> Goto54/1
  Constant20/1 -> Goto53/1
  Constant19/1 -> Goto52/1
  Constant/1 -> Goto51/1
  [v_b] -> Reshape6/1
  Reshape6/1 -> F(X) 9DOF_UVWPQR/4(v_body)
  Reshape5/1 -> F(X) 9DOF_UVWPQR/3(omega_body)
  Reshape4/1 -> F(X) 9DOF_UVWPQR/2(gforce_body)
  [omega_b] -> Reshape5/1
  Reshape3/1 -> F(X) 9DOF_UVWPQR/1(prev_input)
  Reshape2/1 -> Sum2/1
  Reshape/1 -> Sum2/2
  Mux4/1 -> Reshape/1  "y_dot_desired"
  Tuning perturbation7/1 -> Sum13/2
  Tuning perturbation6/1 -> Sum14/2
  Tuning perturbation8/1 -> Sum8/2
  Sum13/1 -> PID Controller7/1
  Sum8/1 -> PID Controller8/1
  Sum14/1 -> PID Controller6/1
  Constant16/1 -> PID Controller7/3
  Constant17/1 -> PID Controller7/2
  Constant14/1 -> PID Controller8/3
  Constant15/1 -> PID Controller8/2
  PID Controller8/1 -> [r_dot_des], Mux5/3
  PID Controller7/1 -> [q_dot_des], Mux5/2
  PID Controller6/1 -> [p_dot_des], Mux5/1
  Tuning perturbation4/1 -> Sum12/2
  Tuning perturbation/1 -> Sum9/2
  Tuning perturbation5/1 -> Sum10/2
  Sum12/1 -> PID Controller4/1
  Sum10/1 -> PID Controller5/1
  Sum9/1 -> PID Controller/1
  Constant7/1 -> PID Controller4/3
  Constant9/1 -> PID Controller/3
  Constant10/1 -> PID Controller/2
  Constant8/1 -> PID Controller4/2
  Constant5/1 -> PID Controller5/3
  Constant6/1 -> PID Controller5/2
  PID Controller5/1 -> [r_ref]
  PID Controller4/1 -> [q_ref]
  PID Controller/1 -> [p_ref]
  Tuning perturbation3/1 -> Sum7/2
  [vz_error] -> Sum7/1
  Sum7/1 -> PID Controller2/1
  Constant3/1 -> PID Controller2/3
  Constant4/1 -> PID Controller2/2
  [gforce_body] -> Reshape4/1
  Earth to body1/1 -> [gforce_body]
  Gravity/1 -> Earth to body1/2
  F(X) 9DOF_UVWPQR/1(fx) -> Reshape2/1
  Mux/1 -> Sum/1
  Demux3/3 -> [r]
  Demux3/2 -> [q]
  Demux3/1 -> [p]
  Demux2/1 -> [phi]
  Demux2/2 -> [theta]
  Demux2/3 -> [psi]
  measurements/1 -> Bus Selector/1
  Bus Selector/1 -> Demux2/1, Sum/2  "<euler>"
  Bus Selector/2 -> Demux3/1, Sum1/1, [omega_b]  "<omega_b>"
  Sum1/1 -> Demux/1
  Sum/1 -> Demux1/1
  Demux/3 -> [r_error]
  Demux/2 -> [q_error]
  Demux/1 -> [p_error]
  Demux1/1 -> [phi_error]
  Demux1/2 -> [theta_error]
  Demux1/3 -> [psi_error]
  trim_control_input/1 -> [trimmed_input]
  [theta_ref] -> Mux/2
  [phi_ref] -> Mux/1
  [psi_ref] -> Mux/3
  Mux2/1 -> Sum1/2
  [q_ref] -> Mux2/2
  [p_ref] -> Mux2/1
  [r_ref] -> Mux2/3
  Bus Selector/3 -> Demux5/1, Sum3/1  "<X_e>"
  Demux5/3 -> [Z_earth]
  Demux5/2 -> [Y_earth]
  Demux5/1 -> [X_earth]
  Demux4/3 -> [z_error]
  Demux4/2 -> [y_error]
  Demux4/1 -> [x_error]
  Mux1/1 -> Sum3/2
  [Yearth_ref] -> Mux1/2
  [Xearth_ref] -> Mux1/1
  [Zearth_ref] -> Mux1/3
  Mux3/1 -> Sum4/1
  Demux7/1 -> [vx_b]
  Demux7/2 -> [vy_b]
  Demux7/3 -> [vz_b]
  Bus Selector/5 -> Demux7/1, Sum4/2, [v_b]  "<V_b>"
  Sum4/1 -> Demux6/1
  Demux6/1 -> [vx_error]
  Demux6/2 -> [vy_error]
  Demux6/3 -> [vz_error]
  [Vy_body_ref] -> Mux3/2
  [Vx_body_ref] -> Mux3/1
  [Vz_body_ref] -> Mux3/3
  Bus Selector/4 -> [DCM], Earth to body/1  "<DCM>"
  Earth to body/1 -> Demux4/1
  Demux8/3 -> [Zearth_ref]
  Demux8/2 -> [Yearth_ref]
  Demux8/1 -> [Xearth_ref]
  earth_ref/1 -> Demux8/1
  [prev_output] -> Demux9/1
  Demux9/1 -> [throttle1_0]
  Demux9/2 -> [eta1_0]
  Demux9/3 -> [gamma1_0]
  Demux9/4 -> [throttle2_0]
  Demux9/5 -> [eta2_0]
  Demux9/6 -> [gamma2_0]
  Demux9/7 -> [throttle3_0]
  Demux9/8 -> [eta3_0]
  Demux9/9 -> [gamma3_0]
  PID Controller10/1 -> [accY_des]
  Tuning perturbation10/1 -> Sum15/2
  [vy_error] -> Sum15/1
  Sum15/1 -> PID Controller10/1
  Constant36/1 -> PID Controller10/3
  Constant37/1 -> PID Controller10/2
  PID Controller11/1 -> [accX_des]
  Tuning perturbation11/1 -> Sum16/2
  [vx_error] -> Sum16/1
  Sum16/1 -> PID Controller11/1
  Constant38/1 -> PID Controller11/3
  Constant39/1 -> PID Controller11/2
  From16/1 -> Sum5/1
  [accX_des] -> Sum17/1
  [accY_des] -> Sum18/1
  [accZ_des] -> Sum19/1
  [p_dot_des] -> Sum20/1
  [q_dot_des] -> Sum21/1
  [r_dot_des] -> Sum22/1
  Constant40/1 -> Sum17/2
  Constant41/1 -> Sum18/2
  Constant42/1 -> Sum19/2
  Constant43/1 -> Sum20/2
  Constant44/1 -> Sum21/2
  Constant45/1 -> Sum22/2
  Sum22/1 -> Mux4/6
  Sum21/1 -> Mux4/5
  Sum20/1 -> Mux4/4
  Sum19/1 -> Mux4/3
  Sum18/1 -> Mux4/2
  Sum17/1 -> Mux4/1
